simulink library "tool"  (R2014b)
settings: Solver=VariableStepAuto  StartTime=0.0  StopTime=10.0  RelTol=1e-3
settings Model: Creator=Rusty Goh  LastModifiedBy=root
settings DataIOCC: LimitDataPoints=off  SaveFormat=Dataset
settings OptimizationCC: UseDivisionForNetSlopeComputation=off  LifeSpan=auto  SimCompilerOptimization=off
settings DebuggingCC: SolverPrmCheckMsg=none  FcnCallInpInsideContextMsg=error  FrameProcessingCompatibilityMsg=error  SFUnexpectedBacktrackingDiag=error  SFNoUnconditionalDefaultTransitionDiag=error
settings HardwareCC: ProdBitPerPointer=64  ProdLargestAtomicFloat=Float  ProdIntDivRoundTo=Zero  ProdEndianess=LittleEndian  ProdWordSize=64  ProdHWDeviceType=Intel->x86-64 (Windows64)
settings ModelReferenceCC: PropagateSignalLabelsOutOfModel=on
settings RTWCC: RTWCompilerOptimization=off
settings GRTTargetCC: TargetLangStandard=C99 (ISO)  GeneratePreprocessorConditionals=Use local settings

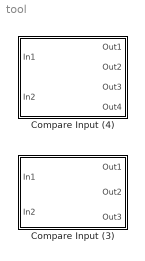
== system tool ==
  Compare Input (3) : Subsystem
  Compare Input (4) : Subsystem

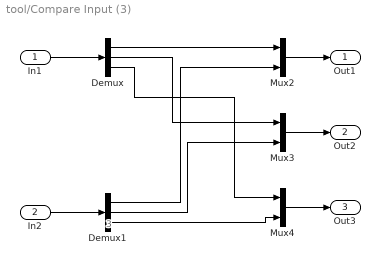
== system tool/Compare Input (3) ==
  note: 3
  In1 : Inport
  In2 : Inport  Port=2
  Demux : Demux  Outputs=3
  Demux1 : Demux  Outputs=3
  Mux2 : Mux  Inputs=2
  Mux3 : Mux  Inputs=2
  Mux4 : Mux  Inputs=2
  Out1 : Outport
  Out2 : Outport  Port=2
  Out3 : Outport  Port=3
  wires:
  Mux4/1 -> Out3/1
  Demux/1 -> Mux2/1
  Demux1/1 -> Mux2/2
  In2/1 -> Demux1/1
  Demux/3 -> Mux4/1
  In1/1 -> Demux/1
  Mux3/1 -> Out2/1
  Demux1/2 -> Mux3/2
  Mux2/1 -> Out1/1
  Demux/2 -> Mux3/1
  Demux1/3 -> Mux4/2

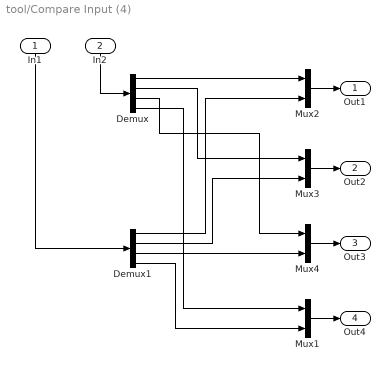
== system tool/Compare Input (4) ==
  In1 : Inport
  In2 : Inport  Port=2
  Demux : Demux
  Demux1 : Demux
  Mux{1..4} (4 alike) : Mux  Inputs=2
  Out1 : Outport
  Out2 : Outport  Port=2
  Out3 : Outport  Port=3
  Out4 : Outport  Port=4
  wires:
  Demux1/2 -> Mux3/2
  Demux/2 -> Mux3/1
  Demux/3 -> Mux4/1
  Demux1/3 -> Mux4/2
  Demux/1 -> Mux2/1
  Mux4/1 -> Out3/1
  Demux1/1 -> Mux2/2
  In1/1 -> Demux1/1
  In2/1 -> Demux/1
  Mux2/1 -> Out1/1
  Mux3/1 -> Out2/1
  Demux/4 -> Mux1/1
  Demux1/4 -> Mux1/2
  Mux1/1 -> Out4/1
